simulink model "exmaple1"  (R2025b)
settings: Solver=VariableStepAuto  StartTime=0.0  StopTime=10.0  RelTol=1e-3
settings Model: Creator=mizula  LastModifiedBy=mizula

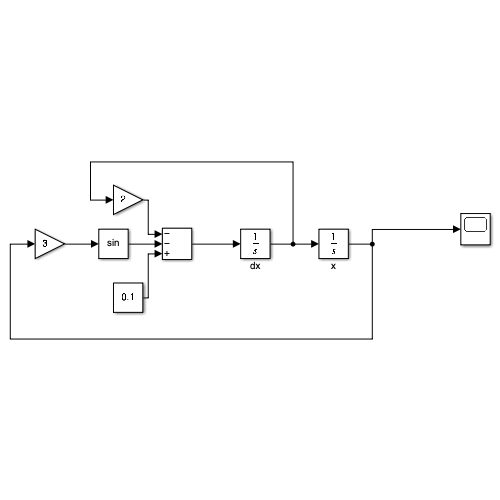
[thumbnail: Simulink's stored preview of the top-level diagram]
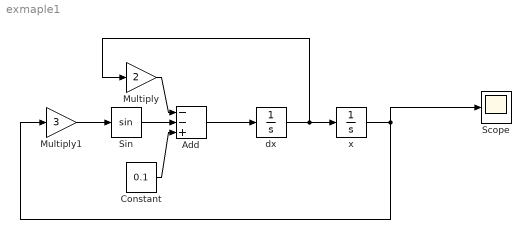
== system exmaple1 ==
  Add : Sum  Inputs=--+
  Constant : Constant  Value=0.1
  Multiply : Gain  Gain=2
  Multiply1 : Gain  Gain=3
  Scope : Scope
      settings: ActiveDisplayYMinimum=-0.41663050668003276  ActiveDisplayYMaximum=0.660474275597785
  Sin : Trigonometry
  dx : Integrator  InitialCondition=2
  x : Integrator
  wires:
  dx/1 -> Multiply/1, x/1
  Add/1 -> dx/1
  Multiply/1 -> Add/1
  Sin/1 -> Add/2
  Multiply1/1 -> Sin/1
  x/1 -> Multiply1/1, Scope/1
  Constant/1 -> Add/3
